simulink model "npc_controller"  (R2022a)
settings: Solver=FixedStepDiscrete  StartTime=0.0  StopTime=20  RelTol=1e-3  EnableMultiTasking=on
values from neighbouring files (symbols this model uses):
  Tsw = 1.5E-5    [param.sldd]
undefined symbols (not defined in the file or in its folder): CAN_O_INT, CANA_BASE, Down, GPTRIP1SEL, GPTRIP2SEL, GPTRIP3SEL, TZ1, TZ2, TZ3, Up
libraries: simulink x153, hdlsllib x90, c2802xlib x34, c2837xDlib x18, c280xlib x12, canmsglib x9, c2838xlib x8, idelinklib_common x3, c2806xlib x2, slpidlib x2, c28004xlib x2, c281xlib x2
(part 30 of 45)

== system npc_controller/CONTROL/STATE-MACHINE/CPU_CONTROL_750_precharge_pfc_ok2/updateSequencePhC/pol_vxn1/neg ==
  note: Note:
      |
      | Function PWM # GPIO # LAUNCHPAD PIN #
      |
      | Synci EPWM1A GPIO0 J4.40
      | EPWM1B GPIO1 J4.39
      |
      | TZ GPIO62 XX
      |
      | a_s1 EPWM6B GPIO11 J8.75
      | a_s2 EPWM7B GPIO13 XX
      | a_s3 EPWM6A GPIO10 J8.76
      | a_s4 EPWM7A GPIO12 XX
      |
      | b_s1 EPWM8B GPIO15 J8.73
      | b_s2 EPWM9B GPIO17 XX
      | b_s3 EPWM8A GPIO14 J8.74
      | b_s4 EPWM9A GPIO16 J4.33
      |
      | c_s1 EPWM10B GPIO19 J1.3
      | c_s2 EPWM11B GPIO21 XX
      | c_s3 EPWM10A GPIO18 J1.4
      | c_s4 EPWM11A GPIO20 XX
  note: EPwm10Regs.AQCSFRC.bit.CSFB = (uint16_T)(0b01);
      | EPwm11Regs.AQCSFRC.bit.CSFB = (uint16_T)(0b00);
      | EPwm10Regs.AQCSFRC.bit.CSFA = (uint16_T)(0b10);
      | EPwm11Regs.AQCSFRC.bit.CSFA = (uint16_T)(0b01);
  note: Note:
      | AQCSFRC
      | 0b00 - disables forced PWM
      | 0b01 - forces PWM to LOW
      | 0b10 - forces PWM to  HIGH
  Action Port : ActionPort  ActionPortLabel=else
  Constant : Constant  Value=2  OutDataTypeStr=uint8  SampleTime=-1
  System Outputs1 : Subsystem  mask(System Outputs){ShowInLibBrowser=0}
      mask prompts: ShowInLibBrowser "Simulink:masks:CustCodeMaskParam1_MP"
      settings: CopyFcn=cccopyfcn(gcb)  OpenFcn=ccopenfcn('System Outputs Function')
      mask Help: eval('feval(''rtwprivate'',''rtwhelpview'',''rtw_sys_outputs_block'')');
      mask Display: disp('System\nOutputs');
  Out1 : Outport
  wires:
  Constant/1 -> Out1/1

== system npc_controller/CONTROL/STATE-MACHINE/CPU_CONTROL_750_precharge_pfc_ok2/updateSequencePhC/pol_vxn1/pos ==
  note: Note:
      | AQCSFRC
      | 0b00 - disables forced PWM
      | 0b01 - forces PWM to LOW
      | 0b10 - forces PWM to  HIGH
  note: Note:
      |
      | Function PWM # GPIO # LAUNCHPAD PIN #
      |
      | Synci EPWM1A GPIO0 J4.40
      | EPWM1B GPIO1 J4.39
      |
      | TZ GPIO62 XX
      |
      | a_s1 EPWM6B GPIO11 J8.75
      | a_s2 EPWM7B GPIO13 XX
      | a_s3 EPWM6A GPIO10 J8.76
      | a_s4 EPWM7A GPIO12 XX
      |
      | b_s1 EPWM8B GPIO15 J8.73
      | b_s2 EPWM9B GPIO17 XX
      | b_s3 EPWM8A GPIO14 J8.74
      | b_s4 EPWM9A GPIO16 J4.33
      |
      | c_s1 EPWM10B GPIO19 J1.3
      | c_s2 EPWM11B GPIO21 XX
      | c_s3 EPWM10A GPIO18 J1.4
      | c_s4 EPWM11A GPIO20 XX
  note: EPwm10Regs.AQCSFRC.bit.CSFB = (uint16_T)(0b01);
      | EPwm11Regs.AQCSFRC.bit.CSFB = (uint16_T)(0b10);
      | EPwm10Regs.AQCSFRC.bit.CSFA = (uint16_T)(0b00);
      | EPwm11Regs.AQCSFRC.bit.CSFA = (uint16_T)(0b01);
  Action Port : ActionPort  ActionPortLabel=elseif(u1 >= 16)
  Constant : Constant  OutDataTypeStr=uint8  SampleTime=-1
  System Outputs1 : Subsystem  mask(System Outputs){ShowInLibBrowser=0}
      mask prompts: ShowInLibBrowser "Simulink:masks:CustCodeMaskParam1_MP"
      settings: CopyFcn=cccopyfcn(gcb)  OpenFcn=ccopenfcn('System Outputs Function')
      mask Help: eval('feval(''rtwprivate'',''rtwhelpview'',''rtw_sys_outputs_block'')');
      mask Display: disp('System\nOutputs');
  Out1 : Outport
  wires:
  Constant/1 -> Out1/1

== system npc_controller/CONTROL/STATE-MACHINE/CPU_CONTROL_750_precharge_pfc_ok2/updateSequencePhC/pol_vxn1/zero ==
  note: Note:
      |
      | Function PWM # GPIO # LAUNCHPAD PIN #
      |
      | Synci EPWM1A GPIO0 J4.40
      | EPWM1B GPIO1 J4.39
      |
      | TZ GPIO62 XX
      |
      | a_s1 EPWM6B GPIO11 J8.75
      | a_s2 EPWM7B GPIO13 XX
      | a_s3 EPWM6A GPIO10 J8.76
      | a_s4 EPWM7A GPIO12 XX
      |
      | b_s1 EPWM8B GPIO15 J8.73
      | b_s2 EPWM9B GPIO17 XX
      | b_s3 EPWM8A GPIO14 J8.74
      | b_s4 EPWM9A GPIO16 J4.33
      |
      | c_s1 EPWM10B GPIO19 J1.3
      | c_s2 EPWM11B GPIO21 XX
      | c_s3 EPWM10A GPIO18 J1.4
      | c_s4 EPWM11A GPIO20 XX
  note: /*Force PWM to LOW*/
      | EPwm10Regs.AQCSFRC.bit.CSFB = (uint16_T)(0b01);
      | EPwm11Regs.AQCSFRC.bit.CSFB = (uint16_T)(0b01);
      | EPwm10Regs.AQCSFRC.bit.CSFA = (uint16_T)(0b01);
      | EPwm11Regs.AQCSFRC.bit.CSFA = (uint16_T)(0b01);
  note: Note:
      | AQCSFRC
      | 0b00 - disables forced PWM
      | 0b01 - forces PWM to LOW
      | 0b10 - forces PWM to  HIGH
  Action Port : ActionPort  ActionPortLabel="if((u1 > -16)  & (u1 < 16))"
  Constant : Constant  Value=0  OutDataTypeStr=uint8  SampleTime=-1
  System Outputs1 : Subsystem  mask(System Outputs){ShowInLibBrowser=0}
      mask prompts: ShowInLibBrowser "Simulink:masks:CustCodeMaskParam1_MP"
      settings: CopyFcn=cccopyfcn(gcb)  OpenFcn=ccopenfcn('System Outputs Function')
      mask Help: eval('feval(''rtwprivate'',''rtwhelpview'',''rtw_sys_outputs_block'')');
      mask Display: disp('System\nOutputs');
  Out1 : Outport
  wires:
  Constant/1 -> Out1/1

== system npc_controller/CONTROL/SVPWM/PLL_Block/SRF_PLL/Integrator ==
  PI Out : Inport  OutDataTypeStr=single
  Accumulation : Subsystem  TreatAsAtomicUnit=on
  Add : Sum  AccumDataTypeStr=single
  Compare To Constant : simulink/Logic and Bit Operations/Compare To Constant  relop=>=  const=2*pi  OutDataTypeStr=boolean
  If : If  IfExpression=u1
  Merge : Merge
  Product : Product  OutDataTypeStr=single
  Reset Integrator : Subsystem  TreatAsAtomicUnit=on
  Ts : Constant  Value=Tsw  OutDataTypeStr=single
  Unit Delay : UnitDelay  SampleTime=-1  HasFrameUpgradeWarning=on
  wt : Outport
  wires:
  Unit Delay/1 -> Add/2, wt/1
  Merge/1 -> Unit Delay/1
  Accumulation/1(Out) -> Merge/2
  Reset Integrator/1(Out) -> Merge/1
  If/2 -> Accumulation/Action
  If/1 -> Reset Integrator/Action
  Compare To Constant/1 -> If/1
  Add/1 -> Compare To Constant/1, Accumulation/1(In1)
  Product/1 -> Add/1
  Ts/1 -> Product/2
  PI Out/1 -> Product/1

== system npc_controller/CONTROL/SVPWM/PLL_Block/SRF_PLL/PI ==
  Vq : Inport
  Ki : Gain  Gain=200
  Kp : Gain  Gain=0.5
  Sum : Sum  Inputs=|++
  Sum1 : Sum  Inputs=+|+
  Ts/2 : Gain  Gain=Tsw/2
  Unit Delay : UnitDelay  SampleTime=-1  HasFrameUpgradeWarning=on
  PI Out : Outport
  wires:
  Sum/1 -> Unit Delay/1, Sum1/2
  Kp/1 -> Sum1/1
  Unit Delay/1 -> Sum/2
  Vq/1 -> Kp/1, Ki/1  "Vq"
  Ki/1 -> Ts/2/1
  Sum1/1 -> PI Out/1
  Ts/2/1 -> Sum/1

== system npc_controller/CONTROL/SVPWM/PLL_Block/SRF_PLL/Subsystem1 ==
  x[n] : Inport
  1 - Lambda : Gain  Gain=1 - 0.98
  Delay : Delay  DelayLength=1
  Gain{,1..7} (8 alike) : Gain  Commented=on  Gain=1/8
  Lambda : Gain  Gain=0.98
  Memory{,1..6} (7 alike) : Memory  Commented=on  InheritSampleTime=on
  Sum{,1..6} (7 alike) : Sum  Commented=on  Inputs=++|
  Sum7 : Sum  Inputs=|++
  y[n] : Outport
  wires:
  Memory/1 -> Memory1/1, Gain1/1
  Memory1/1 -> Memory2/1, Gain2/1
  Memory2/1 -> Memory3/1, Gain3/1
  Gain/1 -> Sum/2
  Gain1/1 -> Sum/1
  Sum/1 -> Sum1/2
  Gain2/1 -> Sum1/1
  Sum1/1 -> Sum2/2
  Gain3/1 -> Sum2/1
  Gain4/1 -> Sum3/1
  Sum2/1 -> Sum3/2
  Memory3/1 -> Memory4/1, Gain4/1
  Memory4/1 -> Memory5/1, Gain5/1
  Sum3/1 -> Sum4/2
  Gain5/1 -> Sum4/1
  Gain6/1 -> Sum5/1
  Sum4/1 -> Sum5/2
  Memory5/1 -> Memory6/1, Gain6/1
  Memory6/1 -> Gain7/1
  Sum5/1 -> Sum6/2
  Gain7/1 -> Sum6/1
  Lambda/1 -> Sum7/2
  x[n]/1 -> 1 - Lambda/1
  1 - Lambda/1 -> Sum7/1
  Delay/1 -> Lambda/1
  Sum7/1 -> Delay/1, y[n]/1

== system npc_controller/CONTROL/SVPWM/PLL_Block/SRF_PLL/abc to dq ==
  note: wt
  note: wt
  note: wt
  a : Inport
  b : Inport  Port=2
  c : Inport  Port=3
  wt : Inport  Port=4
  (wt+120) : Sum  Inputs=|++
  (wt-120) : Sum  Inputs=|+-
  2pi_3 : Constant  Value=2*pi/3
  Add3 : Sum  Inputs=+++
  Cos3 : Trigonometry  Operator=cos
  Cos4 : Trigonometry  Operator=cos
  Cos5 : Trigonometry  Operator=cos
  Product5 : Product
  Product6 : Product
  Product7 : Product
  q1 : Gain  Gain=2/3
  q : Outport
  wires:
  2pi_3/1 -> [ph]
  q1/1 -> q/1
  [c] -> Product7/1
  Add3/1 -> q1/1
  b/1 -> [b]
  Cos5/1 -> Product7/2
  Product5/1 -> Add3/1
  Cos4/1 -> Product6/2
  [b] -> Product6/1
  (wt-120)/1 -> Cos4/1
  [ph] -> (wt-120)/2
  c/1 -> [c]
  Product6/1 -> Add3/2
  (wt+120)/1 -> Cos5/1
  a/1 -> [a]
  Product7/1 -> Add3/3
  [ph] -> (wt+120)/2
  wt/1 -> Cos3/1, (wt-120)/1, (wt+120)/1
  Cos3/1 -> Product5/2
  [a] -> Product5/1

== system npc_controller/CONTROL/SVPWM/PLL_Block/Subsystem/Initialize at Zero Crossing ==
  In1 : Inport
  Trigger : TriggerPort  VariantControl=Variant
  OR : Logic  Operator=OR  IconShape=distinctive  AllPortsSameDT=off  OutDataTypeStr=boolean
  Unit Delay : UnitDelay  SampleTime=-1  HasFrameUpgradeWarning=on
  Out1 : Outport  InitialOutput=0  VectorParamsAs1DForOutWhenUnconnected=off
  wires:
  In1/1 -> OR/1
  Unit Delay/1 -> OR/2
  OR/1 -> Unit Delay/1, Out1/1

== system npc_controller/IDLE_AND_TIMER/codegen/CAN_Task/Rx_Handler/ ProcessMB10 ==
  Action Port : ActionPort  ActionPortLabel=if(u1 == 1)
  All Legs : Subsystem  TreatAsAtomicUnit=on
  Bit Shift : hdlsllib/Logic and Bit Operations/Bit Shift  mode=Shift Right Logical  N=1
  Bitwise AND : simulink/Logic and Bit Operations/Bitwise Operator  logicop=AND  UseBitMask=on  BitMask=hex2dec('01')  BitMaskRealWorld=Stored Integer
  Bitwise AND1 : simulink/Logic and Bit Operations/Bitwise Operator  logicop=AND  UseBitMask=on  BitMask=hex2dec('0E')  BitMaskRealWorld=Stored Integer
  Constant : Constant  Value=10
  Constant1 : Constant  Value=0  OutDataTypeStr=boolean
  Constant10 : Constant  Value=[7:7]
  Constant11 : Constant  Value=[1:1]
  Constant2 : Constant  Value=[0:0]
  Constant3 : Constant  Value=[2:2]
  Constant4 : Constant  Value=[3:3]
  Constant5 : Constant  Value=100
  Constant6 : Constant  Value=[4:4]
  Constant7 : Constant  Value=[5:5]
  Constant8 : Constant
  Constant9 : Constant  Value=[6:6]
  Data Store Read : DataStoreRead  DataStoreName=u8CanDataRx10  IndexOptions=Index vector (dialog)  Indices=1  OutputSizes=1
  Data Store Write1 : DataStoreWrite  DataStoreName=b05_MB10Received  IndexOptions=Index vector (dialog)  Indices=1  OutputSizes=1
  Data Store Write2 : DataStoreWrite  DataStoreName=f32VoutTarget  IndexOptions=Index vector (dialog)  Indices=1  OutputSizes=1
  Data Store Write3 : DataStoreWrite  DataStoreName=f32IoutTarget  IndexOptions=Index vector (dialog)  Indices=1  OutputSizes=1
  Data Store Write4 : DataStoreWrite  DataStoreName=f32V2GPwrTarget  IndexOptions=Index vector (dialog)  Indices=1  OutputSizes=1
  Data Type Conversion{1..2,5..6,9..10} (6 alike) : DataTypeConversion  OutDataTypeStr=uint16  SaturateOnIntegerOverflow=off  RndMeth=Floor
  Data Type Conversion{3..4,7..8,11..12} (6 alike) : DataTypeConversion  OutDataTypeStr=single  SaturateOnIntegerOverflow=off  RndMeth=Floor
  Data Type Conversion13 : DataTypeConversion  OutDataTypeStr=uint8  SaturateOnIntegerOverflow=off  RndMeth=Floor
  Divide : Product  Inputs=*/
  Divide1 : Product  Inputs=*/
  Divide2 : Product  Inputs=*/
  Equal{,1..4} (5 alike) : RelationalOperator  Operator===  OutDataTypeStr=boolean  RndMeth=Simplest  InputSameDT=off
  Frwd : Constant  Value=0xA2
  If : If  IfExpression=u1 == 1
  If1 : If  IfExpression=u1 == 1
  If2 : If  IfExpression=u1 == 1  ElseIfExpressions=u1 == 2, u1 == 3, u1 == 4
  Leg A : Subsystem  TreatAsAtomicUnit=on
  Leg B : Subsystem  TreatAsAtomicUnit=on
  Leg C : Subsystem  TreatAsAtomicUnit=on
  Mode_Cmd : Subsystem  TreatAsAtomicUnit=on
  Multiply1 : Gain  Gain=256
  Multiply2 : Gain  Gain=256
  Multiply3 : Gain  Gain=256
  OR : Logic  Operator=OR  Inputs=5  IconShape=distinctive  AllPortsSameDT=off  OutDataTypeStr=boolean
  Phase Type 1 Phase : Subsystem  TreatAsAtomicUnit=on
  Phase Type 3 Phase : Subsystem  TreatAsAtomicUnit=on
  Rev : Constant  Value=0xA3
  Selector{1..8} (8 alike) : Selector  IndexMode=Zero-based  InputPortWidth=8  IndexOptions=Index vector (port)  Indices=[1 3]  OutputSizes=1
  Sleep : Constant  Value=0xA0
  Stby : Constant  Value=0xA1
  Sum : Sum  Inputs=|++
  Sum1 : Sum  Inputs=|++
  Sum2 : Sum  Inputs=|++
  Test : Constant  Value=0xA4
  wires:
  Constant1/1 -> Data Store Write1/1
  Constant2/1 -> Selector1/2
  Constant3/1 -> Selector2/2
  Constant4/1 -> Selector3/2
  Selector2/1 -> Data Type Conversion1/1
  Data Type Conversion1/1 -> Sum/1
  Selector3/1 -> Data Type Conversion2/1
  Data Type Conversion2/1 -> Multiply1/1
  Multiply1/1 -> Sum/2
  Sum/1 -> Data Type Conversion3/1
  Constant/1 -> Divide/2
  Divide/1 -> Data Type Conversion4/1
  Data Type Conversion3/1 -> Divide/1
  Data Type Conversion4/1 -> Data Store Write2/1
  Data Type Conversion8/1 -> Data Store Write3/1
  Data Type Conversion7/1 -> Divide1/1
  Divide1/1 -> Data Type Conversion8/1
  Constant5/1 -> Divide1/2
  Sum1/1 -> Data Type Conversion7/1
  Multiply2/1 -> Sum1/2
  Data Type Conversion6/1 -> Multiply2/1
  Selector5/1 -> Data Type Conversion6/1
  Data Type Conversion5/1 -> Sum1/1
  Selector4/1 -> Data Type Conversion5/1
  Constant7/1 -> Selector5/2
  Constant6/1 -> Selector4/2
  Constant9/1 -> Selector6/2
  Constant10/1 -> Selector7/2
  Selector6/1 -> Data Type Conversion9/1
  Data Type Conversion9/1 -> Sum2/1
  Selector7/1 -> Data Type Conversion10/1
  Data Type Conversion10/1 -> Multiply3/1
  Multiply3/1 -> Sum2/2
  Sum2/1 -> Data Type Conversion11/1
  Constant8/1 -> Divide2/2
  Divide2/1 -> Data Type Conversion12/1
  Data Type Conversion11/1 -> Divide2/1
  Data Type Conversion12/1 -> Data Store Write4/1
  Stby/1 -> Equal1/2
  OR/1 -> If/1
  Rev/1 -> Equal3/2
  Equal1/1 -> OR/2
  Frwd/1 -> Equal2/2
  Equal2/1 -> OR/3
  Equal3/1 -> OR/4
  Data Type Conversion13/1 -> Mode_Cmd/1(Input)
  Equal/1 -> OR/1
  Sleep/1 -> Equal/2
  If/1 -> Mode_Cmd/Action
  Selector1/1 -> Equal4/1, Data Type Conversion13/1, Equal3/1, Equal2/1, Equal1/1, Equal/1
  Test/1 -> Equal4/2
  Equal4/1 -> OR/5
  Data Store Read/1 -> Selector8/1, Selector6/1, Selector7/1, Selector5/1, Selector4/1, Selector3/1, Selector2/1, Selector1/1
  Constant11/1 -> Selector8/2
  Selector8/1 -> Bitwise AND1/1, Bitwise AND/1
  Bitwise AND/1 -> If1/1
  If1/1 -> Phase Type 1 Phase/Action
  If1/2 -> Phase Type 3 Phase/Action
  Bitwise AND1/1 -> Bit Shift/1
  Bit Shift/1 -> If2/1
  If2/1 -> Leg A/Action
  If2/2 -> Leg B/Action
  If2/4 -> All Legs/Action
  If2/3 -> Leg C/Action

== system npc_controller/IDLE_AND_TIMER/codegen/CAN_Task/Rx_Handler/ProcessMB11 ==
  Action Port : ActionPort  ActionPortLabel=elseif(u2 ==1)
  Constant : Constant  Value=0  OutDataTypeStr=boolean
  Constant1 : Constant  Value=[1:1]
  Constant2 : Constant  Value=[0:0]
  Data Store Read : DataStoreRead  DataStoreName=u8CanDataRx11  IndexOptions=Index vector (dialog)  Indices=1  OutputSizes=1
  Data Store Write1 : DataStoreWrite  DataStoreName=b06_MB11Received  IndexOptions=Index vector (dialog)  Indices=1  OutputSizes=1
  Data Store Write5 : DataStoreWrite  DataStoreName=u8AliveCounter  IndexOptions=Index vector (dialog)  Indices=1  OutputSizes=1
  Data Type Conversion : DataTypeConversion  OutDataTypeStr=uint8  SaturateOnIntegerOverflow=off  RndMeth=Floor
  Data Type Conversion1 : DataTypeConversion  OutDataTypeStr=uint8  SaturateOnIntegerOverflow=off  RndMeth=Floor
  Equal{,1..3} (4 alike) : RelationalOperator  Operator===  OutDataTypeStr=boolean  RndMeth=Simplest  InputSameDT=off
  If : If  IfExpression=u1 == 1
  OR : Logic  Operator=OR  Inputs=4  IconShape=distinctive  AllPortsSameDT=off  OutDataTypeStr=boolean
  Red_Frwd : Constant  Value=0xB2
  Red_Mode_Cmd : Subsystem  TreatAsAtomicUnit=on
  Red_Rev : Constant  Value=0xB3
  Red_Sleep : Constant  Value=0xB0
  Red_Stby : Constant  Value=0xB1
  Selector1 : Selector  IndexMode=Zero-based  InputPortWidth=8  IndexOptions=Index vector (port)  Indices=[1 3]  OutputSizes=1
  Selector2 : Selector  IndexMode=Zero-based  InputPortWidth=8  IndexOptions=Index vector (port)  Indices=[1 3]  OutputSizes=1
  wires:
  Constant/1 -> Data Store Write1/1
  Constant2/1 -> Selector1/2
  Data Type Conversion/1 -> Data Store Write5/1
  Selector1/1 -> Data Type Conversion/1
  Data Store Read/1 -> Selector2/1, Selector1/1
  Constant1/1 -> Selector2/2
  Red_Stby/1 -> Equal1/2
  Selector2/1 -> Equal/1, Data Type Conversion1/1, Equal3/1, Equal2/1, Equal1/1
  Equal2/1 -> OR/3
  Equal/1 -> OR/1
  If/1 -> Red_Mode_Cmd/Action
  OR/1 -> If/1
  Equal3/1 -> OR/4
  Equal1/1 -> OR/2
  Red_Rev/1 -> Equal3/2
  Red_Sleep/1 -> Equal/2
  Red_Frwd/1 -> Equal2/2
  Data Type Conversion1/1 -> Red_Mode_Cmd/1(Input)

== system npc_controller/IDLE_AND_TIMER/codegen/CAN_Task/Rx_Handler/ProcessMB12 ==
  Action Port : ActionPort  ActionPortLabel=elseif( u3==1)
  Constant : Constant  Value=0  OutDataTypeStr=boolean
  Constant2 : Constant  Value=[0:0]
  Data Store Read : DataStoreRead  DataStoreName=u8CanDataRx12  IndexOptions=Index vector (dialog)  Indices=1  OutputSizes=1
  Data Store Write1 : DataStoreWrite  DataStoreName=b07_MB12Received  IndexOptions=Index vector (dialog)  Indices=1  OutputSizes=1
  Debug_Cmd : Subsystem  TreatAsAtomicUnit=on
  Debug_Read : Subsystem  TreatAsAtomicUnit=on
  Debug_Write : Subsystem  TreatAsAtomicUnit=on
  If : If  IfExpression=u1 == 0  ElseIfExpressions=u1 ==1, u1==2
  Selector1 : Selector  IndexMode=Zero-based  InputPortWidth=8  IndexOptions=Index vector (port)  Indices=[1 3]  OutputSizes=1
  wires:
  Constant/1 -> Data Store Write1/1
  Constant2/1 -> Selector1/2
  Data Store Read/1 -> Selector1/1
  Selector1/1 -> If/1
  If/1 -> Debug_Read/Action
  If/2 -> Debug_Write/Action
  If/3 -> Debug_Cmd/Action

== system npc_controller/IDLE_AND_TIMER/codegen/CAN_Task/Tx_Handler/Run Tx Routine ==
  Action Port : ActionPort  ActionPortLabel=if(u1 == u2)
  Constant1 : Constant  Value=0  OutDataTypeStr=uint16
  Data Store Read2 : DataStoreRead  DataStoreName=b01_ReadRequest  IndexOptions=Index vector (dialog)  Indices=1  OutputSizes=1
  Data Store Read3 : DataStoreRead  DataStoreName=b00_DebugEnabled  IndexOptions=Index vector (dialog)  Indices=1  OutputSizes=1
  Data Store Write1 : DataStoreWrite  DataStoreName=u16TxDelayCount  IndexOptions=Index vector (dialog)  Indices=1  OutputSizes=1
  If1 : If  NumInputs=2  IfExpression=u1 == 1 & u2 == 1
  TxReadRequest : Subsystem  TreatAsAtomicUnit=on
  TxStatusData : Subsystem  TreatAsAtomicUnit=on
  wires:
  Constant1/1 -> Data Store Write1/1
  If1/1 -> TxReadRequest/Action
  If1/2 -> TxStatusData/Action
  Data Store Read3/1 -> If1/2
  Data Store Read2/1 -> If1/1

== system npc_controller/IDLE_AND_TIMER/codegen/IDLE/cnt_idle/cnt_idle ==
  Action Port : ActionPort  ActionPortLabel=if(u1 < 6)
  Add : Sum
  Constant : Constant  OutDataTypeStr=uint16
  Data Store Read1 : DataStoreRead  DataStoreName=cnt_idle  IndexOptions=Index vector (dialog)  Indices=1  OutputSizes=1
  Data Store Write : DataStoreWrite  DataStoreName=cnt_idle  IndexOptions=Index vector (dialog)  Indices=1  OutputSizes=1
  wires:
  Data Store Read1/1 -> Add/1
  Add/1 -> Data Store Write/1
  Constant/1 -> Add/2

== system npc_controller/IDLE_AND_TIMER/codegen/IDLE/cnt_idle/cnt_idle_sat ==
  Action Port : ActionPort  ActionPortLabel=else
  Constant : Constant  Value=0  OutDataTypeStr=uint16
  Data Store Write : DataStoreWrite  DataStoreName=cnt_idle  IndexOptions=Index vector (dialog)  Indices=1  OutputSizes=1
  wires:
  Constant/1 -> Data Store Write/1

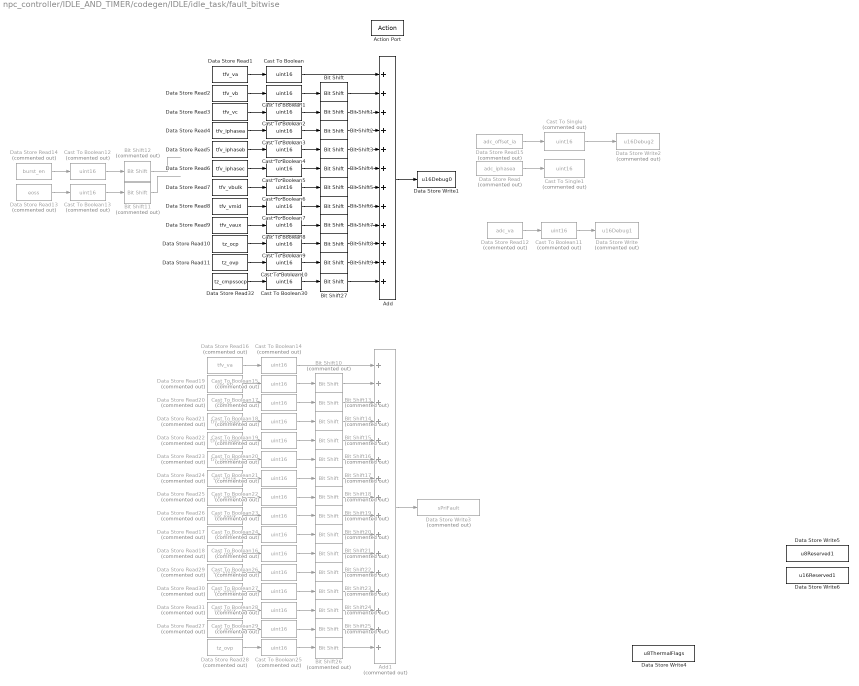
== system npc_controller/IDLE_AND_TIMER/codegen/IDLE/idle_task/fault_bitwise ==
  Action Port : ActionPort  ActionPortLabel=case [ 6 ]:
  Add : Sum  Inputs=++++++++++++
  Add1 : Sum  Commented=on  Inputs=++++++++++++++++
  Bit Shift : hdlsllib/Logic and Bit Operations/Bit Shift  mode=Shift Left Logical  N=1
  Bit Shift1 : hdlsllib/Logic and Bit Operations/Bit Shift  mode=Shift Left Logical  N=2
  Bit Shift10 : hdlsllib/Logic and Bit Operations/Bit Shift  Commented=on  mode=Shift Left Logical  N=1
  Bit Shift11 : hdlsllib/Logic and Bit Operations/Bit Shift  Commented=on  mode=Shift Left Logical  N=11
  Bit Shift12 : hdlsllib/Logic and Bit Operations/Bit Shift  Commented=on  mode=Shift Left Logical  N=10
  Bit Shift13 : hdlsllib/Logic and Bit Operations/Bit Shift  Commented=on  mode=Shift Left Logical  N=2
  Bit Shift14 : hdlsllib/Logic and Bit Operations/Bit Shift  Commented=on  mode=Shift Left Logical  N=3
  Bit Shift15 : hdlsllib/Logic and Bit Operations/Bit Shift  Commented=on  mode=Shift Left Logical  N=4
  Bit Shift16 : hdlsllib/Logic and Bit Operations/Bit Shift  Commented=on  mode=Shift Left Logical  N=5
  Bit Shift17 : hdlsllib/Logic and Bit Operations/Bit Shift  Commented=on  mode=Shift Left Logical  N=6
  Bit Shift18 : hdlsllib/Logic and Bit Operations/Bit Shift  Commented=on  mode=Shift Left Logical  N=7
  Bit Shift19 : hdlsllib/Logic and Bit Operations/Bit Shift  Commented=on  mode=Shift Left Logical  N=8
  Bit Shift2 : hdlsllib/Logic and Bit Operations/Bit Shift  mode=Shift Left Logical  N=3
  Bit Shift20 : hdlsllib/Logic and Bit Operations/Bit Shift  Commented=on  mode=Shift Left Logical  N=9
  Bit Shift21 : hdlsllib/Logic and Bit Operations/Bit Shift  Commented=on  mode=Shift Left Logical  N=10
  Bit Shift22 : hdlsllib/Logic and Bit Operations/Bit Shift  Commented=on  mode=Shift Left Logical  N=11
  Bit Shift23 : hdlsllib/Logic and Bit Operations/Bit Shift  Commented=on  mode=Shift Left Logical  N=12
  Bit Shift24 : hdlsllib/Logic and Bit Operations/Bit Shift  Commented=on  mode=Shift Left Logical  N=13
  Bit Shift25 : hdlsllib/Logic and Bit Operations/Bit Shift  Commented=on  mode=Shift Left Logical  N=14
  Bit Shift26 : hdlsllib/Logic and Bit Operations/Bit Shift  Commented=on  mode=Shift Left Logical  N=15
  Bit Shift27 : hdlsllib/Logic and Bit Operations/Bit Shift  mode=Shift Left Logical  N=11
  Bit Shift3 : hdlsllib/Logic and Bit Operations/Bit Shift  mode=Shift Left Logical  N=4
  Bit Shift4 : hdlsllib/Logic and Bit Operations/Bit Shift  mode=Shift Left Logical  N=5
  Bit Shift5 : hdlsllib/Logic and Bit Operations/Bit Shift  mode=Shift Left Logical  N=6
  Bit Shift6 : hdlsllib/Logic and Bit Operations/Bit Shift  mode=Shift Left Logical  N=7
  Bit Shift7 : hdlsllib/Logic and Bit Operations/Bit Shift  mode=Shift Left Logical  N=8
  Bit Shift8 : hdlsllib/Logic and Bit Operations/Bit Shift  mode=Shift Left Logical  N=9
  Bit Shift9 : hdlsllib/Logic and Bit Operations/Bit Shift  mode=Shift Left Logical  N=10
  Cast To Boolean{,1..10,30} (12 alike) : DataTypeConversion  OutDataTypeStr=uint16  SaturateOnIntegerOverflow=off  RndMeth=Floor
  Cast To Boolean{11..29} (19 alike) : DataTypeConversion  Commented=on  OutDataTypeStr=uint16  SaturateOnIntegerOverflow=off  RndMeth=Floor
  Cast To Single : DataTypeConversion  Commented=on  OutDataTypeStr=uint16  SaturateOnIntegerOverflow=off  RndMeth=Floor
  Cast To Single1 : DataTypeConversion  Commented=on  OutDataTypeStr=uint16  SaturateOnIntegerOverflow=off  RndMeth=Floor
  Data Store Read : DataStoreRead  Commented=on  DataStoreName=adc_iphasea  IndexOptions=Index vector (dialog)  Indices=1  OutputSizes=1
  Data Store Read1 : DataStoreRead  DataStoreName=tfv_va  IndexOptions=Index vector (dialog)  Indices=1  OutputSizes=1
  Data Store Read10 : DataStoreRead  DataStoreName=tz_ocp  IndexOptions=Index vector (dialog)  Indices=1  OutputSizes=1
  Data Store Read11 : DataStoreRead  DataStoreName=tz_ovp  IndexOptions=Index vector (dialog)  Indices=1  OutputSizes=1
  Data Store Read12 : DataStoreRead  Commented=on  DataStoreName=adc_va  IndexOptions=Index vector (dialog)  Indices=1  OutputSizes=1
  Data Store Read13 : DataStoreRead  Commented=on  DataStoreName=eoss  IndexOptions=Index vector (dialog)  Indices=1  OutputSizes=1
  Data Store Read14 : DataStoreRead  Commented=on  DataStoreName=burst_en  IndexOptions=Index vector (dialog)  Indices=1  OutputSizes=1
  Data Store Read15 : DataStoreRead  Commented=on  DataStoreName=adc_offset_ia  IndexOptions=Index vector (dialog)  Indices=1  OutputSizes=1
  Data Store Read16 : DataStoreRead  Commented=on  DataStoreName=tfv_va  IndexOptions=Index vector (dialog)  Indices=1  OutputSizes=1
  Data Store Read17 : DataStoreRead  Commented=on  DataStoreName=tz_ocp  IndexOptions=Index vector (dialog)  Indices=1  OutputSizes=1
  Data Store Read18 : DataStoreRead  Commented=on  DataStoreName=tz_ovp  IndexOptions=Index vector (dialog)  Indices=1  OutputSizes=1
  Data Store Read19 : DataStoreRead  Commented=on  DataStoreName=tfv_vb  IndexOptions=Index vector (dialog)  Indices=1  OutputSizes=1
  Data Store Read2 : DataStoreRead  DataStoreName=tfv_vb  IndexOptions=Index vector (dialog)  Indices=1  OutputSizes=1
  Data Store Read20 : DataStoreRead  Commented=on  DataStoreName=tfv_vc  IndexOptions=Index vector (dialog)  Indices=1  OutputSizes=1
  Data Store Read21 : DataStoreRead  Commented=on  DataStoreName=tfv_iphasea  IndexOptions=Index vector (dialog)  Indices=1  OutputSizes=1
  Data Store Read22 : DataStoreRead  Commented=on  DataStoreName=tfv_iphaseb  IndexOptions=Index vector (dialog)  Indices=1  OutputSizes=1
  Data Store Read23 : DataStoreRead  Commented=on  DataStoreName=tfv_iphasec  IndexOptions=Index vector (dialog)  Indices=1  OutputSizes=1
  Data Store Read24 : DataStoreRead  Commented=on  DataStoreName=tfv_vbulk  IndexOptions=Index vector (dialog)  Indices=1  OutputSizes=1
  Data Store Read25 : DataStoreRead  Commented=on  DataStoreName=tfv_vmid  IndexOptions=Index vector (dialog)  Indices=1  OutputSizes=1
  Data Store Read26 : DataStoreRead  Commented=on  DataStoreName=tfv_vaux  IndexOptions=Index vector (dialog)  Indices=1  OutputSizes=1
  Data Store Read27 : DataStoreRead  Commented=on  DataStoreName=tz_ocp  IndexOptions=Index vector (dialog)  Indices=1  OutputSizes=1
  Data Store Read28 : DataStoreRead  Commented=on  DataStoreName=tz_ovp  IndexOptions=Index vector (dialog)  Indices=1  OutputSizes=1
  Data Store Read29 : DataStoreRead  Commented=on  DataStoreName=tfv_vbulk  IndexOptions=Index vector (dialog)  Indices=1  OutputSizes=1
  Data Store Read3 : DataStoreRead  DataStoreName=tfv_vc  IndexOptions=Index vector (dialog)  Indices=1  OutputSizes=1
  Data Store Read30 : DataStoreRead  Commented=on  DataStoreName=tfv_vmid  IndexOptions=Index vector (dialog)  Indices=1  OutputSizes=1
  Data Store Read31 : DataStoreRead  Commented=on  DataStoreName=tfv_vaux  IndexOptions=Index vector (dialog)  Indices=1  OutputSizes=1
  Data Store Read32 : DataStoreRead  DataStoreName=tz_cmpssocp  IndexOptions=Index vector (dialog)  Indices=1  OutputSizes=1
  Data Store Read4 : DataStoreRead  DataStoreName=tfv_iphasea  IndexOptions=Index vector (dialog)  Indices=1  OutputSizes=1
  Data Store Read5 : DataStoreRead  DataStoreName=tfv_iphaseb  IndexOptions=Index vector (dialog)  Indices=1  OutputSizes=1
  Data Store Read6 : DataStoreRead  DataStoreName=tfv_iphasec  IndexOptions=Index vector (dialog)  Indices=1  OutputSizes=1
  Data Store Read7 : DataStoreRead  DataStoreName=tfv_vbulk  IndexOptions=Index vector (dialog)  Indices=1  OutputSizes=1
  Data Store Read8 : DataStoreRead  DataStoreName=tfv_vmid  IndexOptions=Index vector (dialog)  Indices=1  OutputSizes=1
  Data Store Read9 : DataStoreRead  DataStoreName=tfv_vaux  IndexOptions=Index vector (dialog)  Indices=1  OutputSizes=1
  Data Store Write : DataStoreWrite  Commented=on  DataStoreName=u16Debug1  IndexOptions=Index vector (dialog)  Indices=1  OutputSizes=1
  Data Store Write1 : DataStoreWrite  DataStoreName=u16Debug0  IndexOptions=Index vector (dialog)  Indices=1  OutputSizes=1
  Data Store Write2 : DataStoreWrite  Commented=on  DataStoreName=u16Debug2  IndexOptions=Index vector (dialog)  Indices=1  OutputSizes=1
  Data Store Write3 : DataStoreWrite  Commented=on  DataStoreName=sPriFault  IndexOptions=Index vector (dialog)  Indices=1  OutputSizes=1
  Data Store Write4 : DataStoreWrite  DataStoreName=u8ThermalFlags  IndexOptions=Index vector (dialog)  Indices=1  OutputSizes=1
  Data Store Write5 : DataStoreWrite  DataStoreName=u8Reserved1  IndexOptions=Index vector (dialog)  Indices=1  OutputSizes=1
  Data Store Write6 : DataStoreWrite  DataStoreName=u16Reserved1  IndexOptions=Index vector (dialog)  Indices=1  OutputSizes=1
  wires:
  Add/1 -> Data Store Write1/1
  Data Store Read7/1 -> Cast To Boolean6/1
  Cast To Boolean7/1 -> Bit Shift6/1
  Data Store Read3/1 -> Cast To Boolean2/1
  Cast To Boolean2/1 -> Bit Shift1/1
  Data Store Read1/1 -> Cast To Boolean/1
  Bit Shift5/1 -> Add/7
  Bit Shift/1 -> Add/2
  Data Store Read8/1 -> Cast To Boolean7/1
  Bit Shift3/1 -> Add/5
  Cast To Boolean6/1 -> Bit Shift5/1
  Data Store Read2/1 -> Cast To Boolean1/1
  Bit Shift4/1 -> Add/6
  Bit Shift2/1 -> Add/4
  Cast To Boolean5/1 -> Bit Shift4/1
  Cast To Boolean/1 -> Add/1
  Cast To Boolean1/1 -> Bit Shift/1
  Bit Shift6/1 -> Add/8
  Cast To Boolean3/1 -> Bit Shift2/1
  Cast To Boolean4/1 -> Bit Shift3/1
  Bit Shift1/1 -> Add/3
  Cast To Boolean9/1 -> Bit Shift8/1
  Bit Shift8/1 -> Add/10
  Data Store Read10/1 -> Cast To Boolean9/1
  Data Store Read9/1 -> Cast To Boolean8/1
  Cast To Boolean8/1 -> Bit Shift7/1
  Bit Shift7/1 -> Add/9
  Bit Shift11/1 -> ?
  Bit Shift12/1 -> ?
  Cast To Boolean13/1 -> Bit Shift11/1
  Cast To Boolean12/1 -> Bit Shift12/1
  Data Store Read13/1 -> Cast To Boolean13/1
  Data Store Read14/1 -> Cast To Boolean12/1
  Bit Shift9/1 -> Add/11
  Data Store Read11/1 -> Cast To Boolean10/1
  Cast To Boolean10/1 -> Bit Shift9/1
  Cast To Boolean11/1 -> Data Store Write/1
  Data Store Read12/1 -> Cast To Boolean11/1
  Data Store Read15/1 -> Cast To Single/1
  Data Store Read/1 -> Cast To Single1/1
  Cast To Single/1 -> Data Store Write2/1
  Data Store Read4/1 -> Cast To Boolean3/1
  Data Store Read5/1 -> Cast To Boolean4/1
  Data Store Read6/1 -> Cast To Boolean5/1
  Data Store Read23/1 -> Cast To Boolean20/1
  Data Store Read22/1 -> Cast To Boolean19/1
  Data Store Read21/1 -> Cast To Boolean18/1
  Cast To Boolean16/1 -> Bit Shift21/1
  Data Store Read18/1 -> Cast To Boolean16/1
  Bit Shift21/1 -> Add1/11
  Bit Shift19/1 -> Add1/9
  Cast To Boolean23/1 -> Bit Shift19/1
  Data Store Read26/1 -> Cast To Boolean23/1
  Data Store Read17/1 -> Cast To Boolean24/1
  Bit Shift20/1 -> Add1/10
  Cast To Boolean24/1 -> Bit Shift20/1
  Bit Shift13/1 -> Add1/3
  Cast To Boolean19/1 -> Bit Shift15/1
  Cast To Boolean18/1 -> Bit Shift14/1
  Bit Shift18/1 -> Add1/8
  Cast To Boolean15/1 -> Bit Shift10/1
  Cast To Boolean14/1 -> Add1/1
  Cast To Boolean20/1 -> Bit Shift16/1
  Bit Shift14/1 -> Add1/4
  Bit Shift16/1 -> Add1/6
  Data Store Read19/1 -> Cast To Boolean15/1
  Cast To Boolean21/1 -> Bit Shift17/1
  Bit Shift15/1 -> Add1/5
  Data Store Read25/1 -> Cast To Boolean22/1
  Bit Shift10/1 -> Add1/2
  Bit Shift17/1 -> Add1/7
  Data Store Read16/1 -> Cast To Boolean14/1
  Cast To Boolean17/1 -> Bit Shift13/1
  Data Store Read20/1 -> Cast To Boolean17/1
  Cast To Boolean22/1 -> Bit Shift18/1
  Data Store Read24/1 -> Cast To Boolean21/1
  Data Store Read29/1 -> Cast To Boolean26/1
  Cast To Boolean27/1 -> Bit Shift23/1
  Bit Shift22/1 -> Add1/12
  Data Store Read30/1 -> Cast To Boolean27/1
  Cast To Boolean26/1 -> Bit Shift22/1
  Bit Shift23/1 -> Add1/13
  Cast To Boolean29/1 -> Bit Shift25/1
  Bit Shift25/1 -> Add1/15
  Data Store Read27/1 -> Cast To Boolean29/1
  Data Store Read31/1 -> Cast To Boolean28/1
  Cast To Boolean28/1 -> Bit Shift24/1
  Bit Shift24/1 -> Add1/14
  Bit Shift26/1 -> Add1/16
  Data Store Read28/1 -> Cast To Boolean25/1
  Cast To Boolean25/1 -> Bit Shift26/1
  Add1/1 -> Data Store Write3/1
  Data Store Read32/1 -> Cast To Boolean30/1
  Cast To Boolean30/1 -> Bit Shift27/1
  Bit Shift27/1 -> Add/12

== system npc_controller/IDLE_AND_TIMER/codegen/IDLE/idle_task/get_adc_tmp_mux ==
  Action Port : ActionPort  ActionPortLabel=case [ 5 ]:
  Data Store Read : DataStoreRead  DataStoreName=cnt_tmp_mux  IndexOptions=Index vector (dialog)  Indices=1  OutputSizes=1
  Data Store Read1 : DataStoreRead  DataStoreName=adc_temp_mux  IndexOptions=Index vector (dialog)  Indices=1  OutputSizes=1
  Switch Case : SwitchCase  CaseConditions={0, 1, 2, 3}
  get_tmp_mux_inlet : Subsystem  TreatAsAtomicUnit=on
  get_tmp_mux_npca : Subsystem  TreatAsAtomicUnit=on
  get_tmp_mux_npcb : Subsystem  TreatAsAtomicUnit=on
  get_tmp_mux_npcc : Subsystem  TreatAsAtomicUnit=on
  wires:
  Data Store Read/1 -> Switch Case/1
  Switch Case/1 -> get_tmp_mux_npca/Action
  Switch Case/2 -> get_tmp_mux_npcb/Action
  Switch Case/3 -> get_tmp_mux_npcc/Action
  Switch Case/4 -> get_tmp_mux_inlet/Action
  Data Store Read1/1 -> get_tmp_mux_npcb/1(In1), get_tmp_mux_npca/1(In1), get_tmp_mux_npcc/1(In1), get_tmp_mux_inlet/1(In1)

== system npc_controller/IDLE_AND_TIMER/codegen/IDLE/idle_task/hkeep ==
  note: prot and status
  Action Port : ActionPort  ActionPortLabel=case [ 2 ]:
  Function-Call Generator1 : simulink/Ports & Subsystems/Function-Call Generator  sample_time=-1  numberOfIterations=1  DisallowWideOutput=off
  Function-Call Split3 : FunctionCallSplit  NumOutputPorts=2
  tfv : Subsystem  TreatAsAtomicUnit=on
      settings: RTWSystemCode=Inline
  tz : Subsystem  TreatAsAtomicUnit=on
      settings: RTWSystemCode=Inline
  tz1 : Subsystem  Commented=on  TreatAsAtomicUnit=on
      settings: RTWSystemCode=Inline
  wires:
  Function-Call Split3/1 -> tz/Trigger
  Function-Call Split3/2 -> tfv/Trigger
  Function-Call Generator1/1 -> Function-Call Split3/1

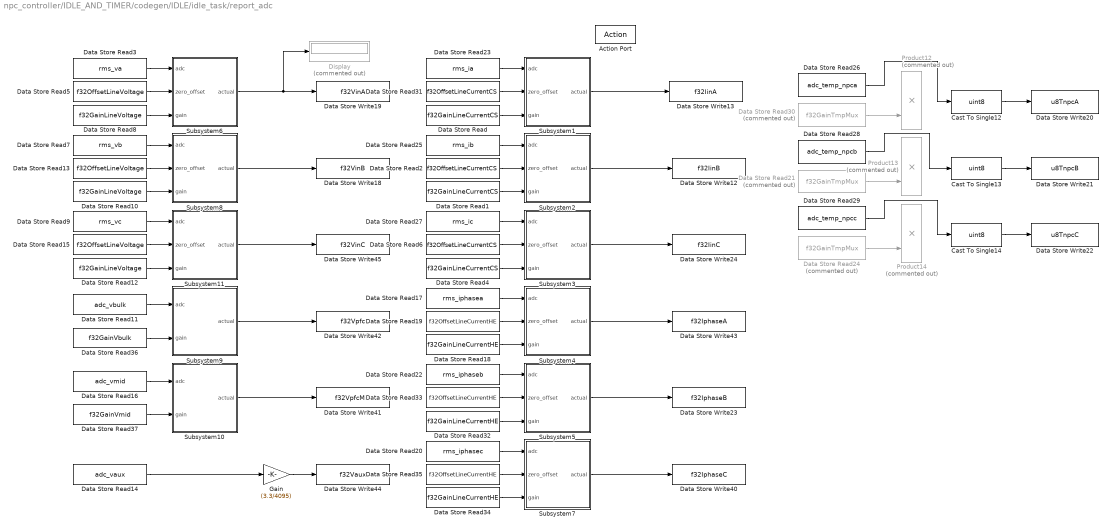
== system npc_controller/IDLE_AND_TIMER/codegen/IDLE/idle_task/report_adc ==
  Action Port : ActionPort  ActionPortLabel=case [ 3 ]:
  Cast To Single12 : DataTypeConversion  OutDataTypeStr=uint8  SaturateOnIntegerOverflow=off  RndMeth=Floor
  Cast To Single13 : DataTypeConversion  OutDataTypeStr=uint8  SaturateOnIntegerOverflow=off  RndMeth=Floor
  Cast To Single14 : DataTypeConversion  OutDataTypeStr=uint8  SaturateOnIntegerOverflow=off  RndMeth=Floor
  Data Store Read : DataStoreRead  DataStoreName=f32GainLineCurrentCS  IndexOptions=Index vector (dialog)  Indices=1  OutputSizes=1
  Data Store Read1 : DataStoreRead  DataStoreName=f32GainLineCurrentCS  IndexOptions=Index vector (dialog)  Indices=1  OutputSizes=1
  Data Store Read10 : DataStoreRead  DataStoreName=f32GainLineVoltage  IndexOptions=Index vector (dialog)  Indices=1  OutputSizes=1
  Data Store Read11 : DataStoreRead  DataStoreName=adc_vbulk  IndexOptions=Index vector (dialog)  Indices=1  OutputSizes=1
  Data Store Read12 : DataStoreRead  DataStoreName=f32GainLineVoltage  IndexOptions=Index vector (dialog)  Indices=1  OutputSizes=1
  Data Store Read13 : DataStoreRead  DataStoreName=f32OffsetLineVoltage  IndexOptions=Index vector (dialog)  Indices=1  OutputSizes=1
  Data Store Read14 : DataStoreRead  DataStoreName=adc_vaux  IndexOptions=Index vector (dialog)  Indices=1  OutputSizes=1
  Data Store Read15 : DataStoreRead  DataStoreName=f32OffsetLineVoltage  IndexOptions=Index vector (dialog)  Indices=1  OutputSizes=1
  Data Store Read16 : DataStoreRead  DataStoreName=adc_vmid  IndexOptions=Index vector (dialog)  Indices=1  OutputSizes=1
  Data Store Read17 : DataStoreRead  DataStoreName=rms_iphasea  IndexOptions=Index vector (dialog)  Indices=1  OutputSizes=1
  Data Store Read18 : DataStoreRead  DataStoreName=f32GainLineCurrentHE  IndexOptions=Index vector (dialog)  Indices=1  OutputSizes=1
  Data Store Read19 : DataStoreRead  DataStoreName=f32OffsetLineCurrentHE  IndexOptions=Index vector (dialog)  Indices=1  OutputSizes=1
  Data Store Read2 : DataStoreRead  DataStoreName=f32OffsetLineCurrentCS  IndexOptions=Index vector (dialog)  Indices=1  OutputSizes=1
  Data Store Read20 : DataStoreRead  DataStoreName=rms_iphasec  IndexOptions=Index vector (dialog)  Indices=1  OutputSizes=1
  Data Store Read21 : DataStoreRead  Commented=on  DataStoreName=f32GainTmpMux  IndexOptions=Index vector (dialog)  Indices=1  OutputSizes=1
  Data Store Read22 : DataStoreRead  DataStoreName=rms_iphaseb  IndexOptions=Index vector (dialog)  Indices=1  OutputSizes=1
  Data Store Read23 : DataStoreRead  DataStoreName=rms_ia  IndexOptions=Index vector (dialog)  Indices=1  OutputSizes=1
  Data Store Read24 : DataStoreRead  Commented=on  DataStoreName=f32GainTmpMux  IndexOptions=Index vector (dialog)  Indices=1  OutputSizes=1
  Data Store Read25 : DataStoreRead  DataStoreName=rms_ib  IndexOptions=Index vector (dialog)  Indices=1  OutputSizes=1
  Data Store Read26 : DataStoreRead  DataStoreName=adc_temp_npca  IndexOptions=Index vector (dialog)  Indices=1  OutputSizes=1
  Data Store Read27 : DataStoreRead  DataStoreName=rms_ic  IndexOptions=Index vector (dialog)  Indices=1  OutputSizes=1
  Data Store Read28 : DataStoreRead  DataStoreName=adc_temp_npcb  IndexOptions=Index vector (dialog)  Indices=1  OutputSizes=1
  Data Store Read29 : DataStoreRead  DataStoreName=adc_temp_npcc  IndexOptions=Index vector (dialog)  Indices=1  OutputSizes=1
  Data Store Read3 : DataStoreRead  DataStoreName=rms_va  IndexOptions=Index vector (dialog)  Indices=1  OutputSizes=1
  Data Store Read30 : DataStoreRead  Commented=on  DataStoreName=f32GainTmpMux  IndexOptions=Index vector (dialog)  Indices=1  OutputSizes=1
  Data Store Read31 : DataStoreRead  DataStoreName=f32OffsetLineCurrentCS  IndexOptions=Index vector (dialog)  Indices=1  OutputSizes=1
  Data Store Read32 : DataStoreRead  DataStoreName=f32GainLineCurrentHE  IndexOptions=Index vector (dialog)  Indices=1  OutputSizes=1
  Data Store Read33 : DataStoreRead  DataStoreName=f32OffsetLineCurrentHE  IndexOptions=Index vector (dialog)  Indices=1  OutputSizes=1
  Data Store Read34 : DataStoreRead  DataStoreName=f32GainLineCurrentHE  IndexOptions=Index vector (dialog)  Indices=1  OutputSizes=1
  Data Store Read35 : DataStoreRead  DataStoreName=f32OffsetLineCurrentHE  IndexOptions=Index vector (dialog)  Indices=1  OutputSizes=1
  Data Store Read36 : DataStoreRead  DataStoreName=f32GainVbulk  IndexOptions=Index vector (dialog)  Indices=1  OutputSizes=1
  Data Store Read37 : DataStoreRead  DataStoreName=f32GainVmid  IndexOptions=Index vector (dialog)  Indices=1  OutputSizes=1
  Data Store Read4 : DataStoreRead  DataStoreName=f32GainLineCurrentCS  IndexOptions=Index vector (dialog)  Indices=1  OutputSizes=1
  Data Store Read5 : DataStoreRead  DataStoreName=f32OffsetLineVoltage  IndexOptions=Index vector (dialog)  Indices=1  OutputSizes=1
  Data Store Read6 : DataStoreRead  DataStoreName=f32OffsetLineCurrentCS  IndexOptions=Index vector (dialog)  Indices=1  OutputSizes=1
  Data Store Read7 : DataStoreRead  DataStoreName=rms_vb  IndexOptions=Index vector (dialog)  Indices=1  OutputSizes=1
  Data Store Read8 : DataStoreRead  DataStoreName=f32GainLineVoltage  IndexOptions=Index vector (dialog)  Indices=1  OutputSizes=1
  Data Store Read9 : DataStoreRead  DataStoreName=rms_vc  IndexOptions=Index vector (dialog)  Indices=1  OutputSizes=1
  Data Store Write12 : DataStoreWrite  DataStoreName=f32IinB  IndexOptions=Index vector (dialog)  Indices=1  OutputSizes=1
  Data Store Write13 : DataStoreWrite  DataStoreName=f32IinA  IndexOptions=Index vector (dialog)  Indices=1  OutputSizes=1
  Data Store Write18 : DataStoreWrite  DataStoreName=f32VinB  IndexOptions=Index vector (dialog)  Indices=1  OutputSizes=1
  Data Store Write19 : DataStoreWrite  DataStoreName=f32VinA  IndexOptions=Index vector (dialog)  Indices=1  OutputSizes=1
  Data Store Write20 : DataStoreWrite  DataStoreName=u8TnpcA  IndexOptions=Index vector (dialog)  Indices=1  OutputSizes=1
  Data Store Write21 : DataStoreWrite  DataStoreName=u8TnpcB  IndexOptions=Index vector (dialog)  Indices=1  OutputSizes=1
  Data Store Write22 : DataStoreWrite  DataStoreName=u8TnpcC  IndexOptions=Index vector (dialog)  Indices=1  OutputSizes=1
  Data Store Write23 : DataStoreWrite  DataStoreName=f32IphaseB  IndexOptions=Index vector (dialog)  Indices=1  OutputSizes=1
  Data Store Write24 : DataStoreWrite  DataStoreName=f32IinC  IndexOptions=Index vector (dialog)  Indices=1  OutputSizes=1
  Data Store Write40 : DataStoreWrite  DataStoreName=f32IphaseC  IndexOptions=Index vector (dialog)  Indices=1  OutputSizes=1
  Data Store Write41 : DataStoreWrite  DataStoreName=f32VpfcMid  IndexOptions=Index vector (dialog)  Indices=1  OutputSizes=1
  Data Store Write42 : DataStoreWrite  DataStoreName=f32Vpfc  IndexOptions=Index vector (dialog)  Indices=1  OutputSizes=1
  Data Store Write43 : DataStoreWrite  DataStoreName=f32IphaseA  IndexOptions=Index vector (dialog)  Indices=1  OutputSizes=1
  Data Store Write44 : DataStoreWrite  DataStoreName=f32Vaux  IndexOptions=Index vector (dialog)  Indices=1  OutputSizes=1
  Data Store Write45 : DataStoreWrite  DataStoreName=f32VinC  IndexOptions=Index vector (dialog)  Indices=1  OutputSizes=1
  Display : Display  Commented=on
  Gain : Gain  Gain=(3.3/4095)  ParamDataTypeStr=single  OutDataTypeStr=single
  Product12 : Product  Commented=on  OutDataTypeStr=single
  Product13 : Product  Commented=on  OutDataTypeStr=single
  Product14 : Product  Commented=on  OutDataTypeStr=single
  Subsystem1 : Subsystem
  Subsystem10 : Subsystem
  Subsystem11 : Subsystem
  Subsystem2 : Subsystem
  Subsystem3 : Subsystem
  Subsystem4 : Subsystem
  Subsystem5 : Subsystem
  Subsystem6 : Subsystem
  Subsystem7 : Subsystem
  Subsystem8 : Subsystem
  Subsystem9 : Subsystem
  wires:
  Data Store Read14/1 -> Gain/1
  Cast To Single13/1 -> Data Store Write21/1
  Cast To Single14/1 -> Data Store Write22/1
  Cast To Single12/1 -> Data Store Write20/1
  Data Store Read30/1 -> Product12/2
  Data Store Read21/1 -> Product13/2
  Data Store Read24/1 -> Product14/2
  Data Store Read25/1 -> Subsystem2/1(adc)
  Data Store Read27/1 -> Subsystem3/1(adc)
  Data Store Read17/1 -> Subsystem4/1(adc)
  Data Store Read22/1 -> Subsystem5/1(adc)
  Data Store Read20/1 -> Subsystem7/1(adc)
  Data Store Read2/1 -> Subsystem2/2(zero_offset)
  Data Store Read1/1 -> Subsystem2/3(gain)
  Data Store Read6/1 -> Subsystem3/2(zero_offset)
  Data Store Read4/1 -> Subsystem3/3(gain)
  Data Store Read19/1 -> Subsystem4/2(zero_offset)
  Data Store Read18/1 -> Subsystem4/3(gain)
  Data Store Read32/1 -> Subsystem5/3(gain)
  Data Store Read33/1 -> Subsystem5/2(zero_offset)
  Data Store Read35/1 -> Subsystem7/2(zero_offset)
  Data Store Read34/1 -> Subsystem7/3(gain)
  Data Store Read7/1 -> Subsystem8/1(adc)
  Data Store Read9/1 -> Subsystem11/1(adc)
  Data Store Read11/1 -> Subsystem9/1(adc)
  Data Store Read16/1 -> Subsystem10/1(adc)
  Data Store Read15/1 -> Subsystem11/2(zero_offset)
  Data Store Read12/1 -> Subsystem11/3(gain)
  Data Store Read36/1 -> Subsystem9/2(gain)
  Data Store Read37/1 -> Subsystem10/2(gain)
  Gain/1 -> Data Store Write44/1
  Data Store Read5/1 -> Subsystem6/2(zero_offset)
  Data Store Read8/1 -> Subsystem6/3(gain)
  Data Store Read/1 -> Subsystem1/3(gain)
  Data Store Read31/1 -> Subsystem1/2(zero_offset)
  Data Store Read10/1 -> Subsystem8/3(gain)
  Data Store Read13/1 -> Subsystem8/2(zero_offset)
  Data Store Read26/1 -> Cast To Single12/1
  Data Store Read28/1 -> Cast To Single13/1
  Data Store Read29/1 -> Cast To Single14/1
  Subsystem8/1(actual) -> Data Store Write18/1
  Subsystem11/1(actual) -> Data Store Write45/1
  Subsystem10/1(actual) -> Data Store Write41/1
  Subsystem1/1(actual) -> Data Store Write13/1
  Subsystem2/1(actual) -> Data Store Write12/1
  Data Store Read23/1 -> Subsystem1/1(adc)
  Subsystem9/1(actual) -> Data Store Write42/1
  Subsystem3/1(actual) -> Data Store Write24/1
  Subsystem4/1(actual) -> Data Store Write43/1
  Subsystem5/1(actual) -> Data Store Write23/1
  Subsystem7/1(actual) -> Data Store Write40/1
  Subsystem6/1(actual) -> Display/1, Data Store Write19/1
  Data Store Read3/1 -> Subsystem6/1(adc)
